simulink model "SURVEY_Simulations"  (R2021b)
settings: Solver=ode4  StartTime=0.0  StopTime=60  FixedStep=1e-3  RelTol=1e-3
(part 1 of 2)
settings Model: Creator=hellb  LastModifiedBy=hellb
settings SolverCC: ZeroCrossAlgorithm=Adaptive
settings DebuggingCC: IgnoredZcDiagnostic=none

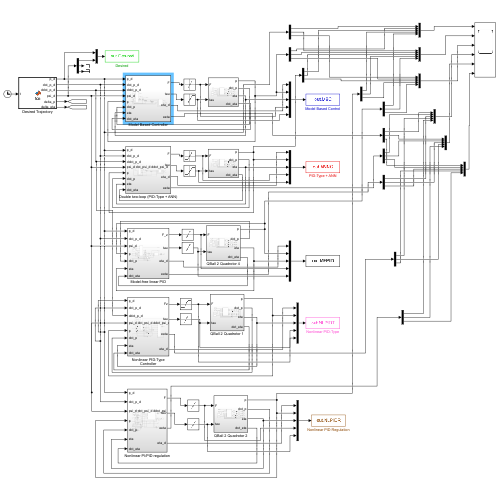
[thumbnail: Simulink's stored preview of the top-level diagram]
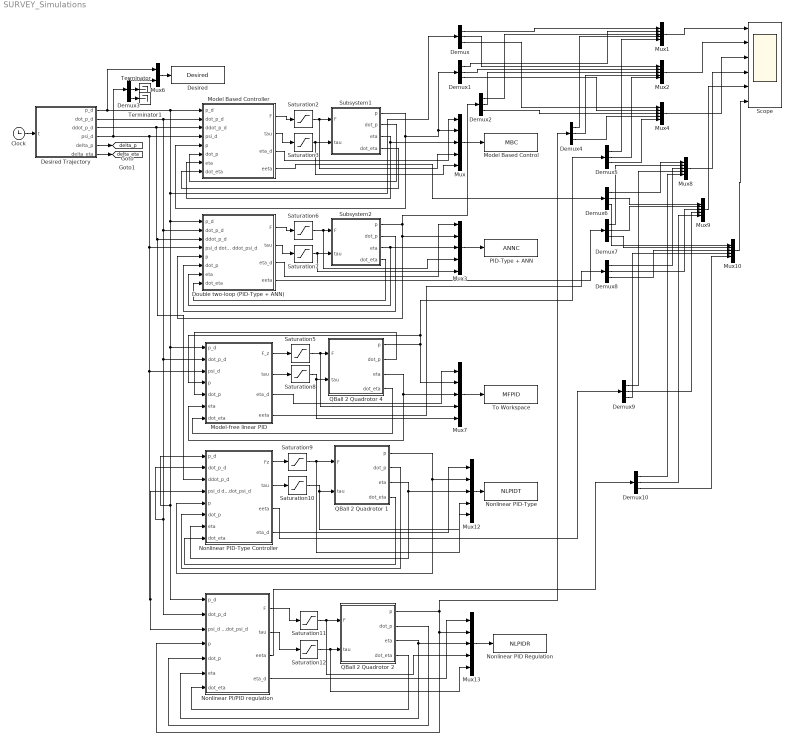
== system SURVEY_Simulations ==
  Clock : Clock
  Demux{,1..10} (11 alike) : Demux  Outputs=3
  Desired : ToWorkspace  VariableName=Desired  SaveFormat=Structure With Time  SampleTime=-1
  Desired Trajectory : MATLAB Function  TreatAsAtomicUnit=on
  Double two-loop (PID-Type + ANN) : Subsystem
  Model Based Control : ToWorkspace  VariableName=MBC  SaveFormat=Structure With Time  SampleTime=-1
  Model Based Controller : Subsystem
  Model-free linear PID : Subsystem
  Mux{,1..4,7..10,12..13} (11 alike) : Mux  Inputs=5
  Mux6 : Mux  Inputs=2
  Nonlinear PI/PID regulation : Subsystem
  Nonlinear PID Regulation : ToWorkspace  VariableName=NLPIDR  SaveFormat=Structure With Time  SampleTime=-1
  Nonlinear PID-Type : ToWorkspace  VariableName=NLPIDT  SaveFormat=Structure With Time  SampleTime=-1
  Nonlinear PID-Type Controller : Subsystem
  PID-Type + ANN : ToWorkspace  VariableName=ANNC  SaveFormat=Structure With Time  SampleTime=-1
  QBall 2 Quadrotor 1 : Subsystem
  QBall 2 Quadrotor 2 : Subsystem
  QBall 2 Quadrotor 4 : Subsystem
  Saturation{3,7..8,10,12} (5 alike) : Saturate  UpperLimit=1.72  LowerLimit=-1.72
  Saturation{2,5..6,9,11} (5 alike) : Saturate  UpperLimit=34.4  LowerLimit=0
  Scope : Scope  NumInputPorts=6
  Subsystem1 : Subsystem
  Subsystem2 : Subsystem
  Terminator : Terminator
  Terminator1 : Terminator
  To Workspace : ToWorkspace  VariableName=MFPID  SaveFormat=Structure With Time  SampleTime=-1
  tag scope: delta_eta=global, delta_p=global
  wires:
  Demux1/3 -> Mux4/2
  Demux3/2 -> Terminator/1
  Subsystem1/2(dot_p) -> Model Based Controller/6(dot_p)
  Demux3/1 -> Mux6/2
  Demux4/3 -> Mux4/4
  Demux4/1 -> Mux1/4
  Demux4/2 -> Mux2/4
  Demux3/3 -> Terminator1/1
  Desired Trajectory/2(dot_p_d) -> Nonlinear PI/PID regulation/2(dot_p_d), Nonlinear PID-Type Controller/2(dot_p_d), Model-free linear PID/2(dot_p_d), Double two-loop (PID-Type + ANN)/2(dot_p_d), Model Based Controller/2(dot_p_d)
  Demux1/2 -> Mux2/2
  Mux6/1 -> Desired/1
  Subsystem2/1(p) -> Demux2/1, Mux3/2, Double two-loop (PID-Type + ANN)/5(p)
  Desired Trajectory/5(delta_p) -> [delta_p]
  Demux/2 -> Mux2/1
  Mux3/1 -> PID-Type + ANN/1
  Mux4/1 -> Scope/3
  Demux2/3 -> Mux4/3
  Desired Trajectory/4(psi_d) -> Nonlinear PI/PID regulation/3(psi_d dot_psi_d ddot_psi_d), Nonlinear PID-Type Controller/4(psi_d dot_psi_d ddot_psi_d), Model-free linear PID/3(psi_d), Double two-loop (PID-Type + ANN)/4(psi_d dot_psi_d ddot_psi_d), Model Based Controller/4(psi_d), Demux3/1
  Double two-loop (PID-Type + ANN)/1(F) -> Saturation6/1
  Model Based Controller/3(eta_d) -> Mux/1
  Mux1/1 -> Scope/1
  Demux/1 -> Mux1/1
  Demux2/2 -> Mux2/3
  Demux2/1 -> Mux1/3
  Model Based Controller/2(tau) -> Saturation3/1
  Desired Trajectory/1(p_d) -> Nonlinear PI/PID regulation/1(p_d), Nonlinear PID-Type Controller/1(p_d), Model-free linear PID/1(p_d), Double two-loop (PID-Type + ANN)/1(p_d), Demux/1, Model Based Controller/1(p_d), Mux6/1
  Subsystem1/1(p) -> Model Based Controller/5(p), Demux1/1, Mux/2
  Subsystem1/4(dot_eta) -> Model Based Controller/8(dot_eta)
  Saturation7/1 -> Subsystem2/2(tau), Mux3/5
  Demux1/1 -> Mux1/2
  Saturation6/1 -> Subsystem2/1(F), Mux3/4
  Subsystem2/2(dot_p) -> Double two-loop (PID-Type + ANN)/6(dot_p)
  Mux/1 -> Model Based Control/1
  Desired Trajectory/3(ddot_p_d) -> Nonlinear PID-Type Controller/3(ddot_p_d), Double two-loop (PID-Type + ANN)/3(ddot_p_d), Model Based Controller/3(ddot_p_d)
  Subsystem1/3(eta) -> Mux/3, Model Based Controller/7(eta)
  Demux/3 -> Mux4/1
  Model Based Controller/1(F) -> Saturation2/1
  Double two-loop (PID-Type + ANN)/3(eta_d) -> Mux3/1
  Double two-loop (PID-Type + ANN)/2(tau) -> Saturation7/1
  Mux2/1 -> Scope/2
  Saturation3/1 -> Mux/5, Subsystem1/2(tau)
  Subsystem2/3(eta) -> Mux3/3, Double two-loop (PID-Type + ANN)/7(eta)
  Desired Trajectory/6(delta_eta) -> [delta_eta]
  Clock/1 -> Desired Trajectory/1(t)
  Subsystem2/4(dot_eta) -> Double two-loop (PID-Type + ANN)/8(dot_eta)
  Model-free linear PID/1(F_z) -> Saturation5/1
  Saturation5/1 -> Mux7/4, QBall 2 Quadrotor 4/1(F)
  QBall 2 Quadrotor 4/4(dot_eta) -> Model-free linear PID/7(dot_eta)
  QBall 2 Quadrotor 4/3(eta) -> Mux7/3, Model-free linear PID/6(eta)
  QBall 2 Quadrotor 4/2(dot_p) -> Model-free linear PID/5(dot_p)
  QBall 2 Quadrotor 4/1(p) -> Mux7/2, Demux5/1, Model-free linear PID/4(p)
  Saturation2/1 -> Mux/4, Subsystem1/1(F)
  Saturation10/1 -> Mux12/5, QBall 2 Quadrotor 1/2(tau)
  Saturation9/1 -> QBall 2 Quadrotor 1/1(F), Mux12/4
  Nonlinear PID-Type Controller/1(Fz) -> Saturation9/1
  Nonlinear PID-Type Controller/2(tau) -> Saturation10/1
  Demux5/1 -> Mux1/5
  Demux5/2 -> Mux2/5
  Demux5/3 -> Mux4/5
  QBall 2 Quadrotor 1/1(p) -> Mux12/2, Nonlinear PID-Type Controller/5(p)
  QBall 2 Quadrotor 1/2(dot_p) -> Nonlinear PID-Type Controller/6(dot_p)
  QBall 2 Quadrotor 1/3(eta) -> Nonlinear PID-Type Controller/7(eta), Mux12/3
  QBall 2 Quadrotor 1/4(dot_eta) -> Nonlinear PID-Type Controller/8(dot_eta)
  Saturation11/1 -> Mux13/4, QBall 2 Quadrotor 2/1(F)
  Saturation12/1 -> Mux13/5, QBall 2 Quadrotor 2/2(tau)
  Nonlinear PI/PID regulation/1(F) -> Saturation11/1
  Nonlinear PI/PID regulation/2(tau) -> Saturation12/1
  QBall 2 Quadrotor 2/1(p) -> Mux13/2, Nonlinear PI/PID regulation/4(p), Demux4/1
  QBall 2 Quadrotor 2/4(dot_eta) -> Nonlinear PI/PID regulation/7(dot_eta)
  QBall 2 Quadrotor 2/3(eta) -> Mux13/3, Nonlinear PI/PID regulation/6(eta)
  QBall 2 Quadrotor 2/2(dot_p) -> Nonlinear PI/PID regulation/5(dot_p)
  Mux9/1 -> Scope/5
  Mux8/1 -> Scope/4
  Mux10/1 -> Scope/6
  Demux6/1 -> Mux8/1
  Demux6/2 -> Mux9/1
  Demux6/3 -> Mux10/1
  Model Based Controller/4(eeta) -> Demux6/1
  Demux7/1 -> Mux8/2
  Demux7/2 -> Mux9/2
  Demux7/3 -> Mux10/2
  Double two-loop (PID-Type + ANN)/4(eeta) -> Demux7/1
  Demux8/1 -> Mux8/3
  Demux8/2 -> Mux9/3
  Demux8/3 -> Mux10/3
  Nonlinear PID-Type Controller/3(eeta) -> Demux9/1
  Demux9/1 -> Mux8/4
  Demux9/2 -> Mux9/4
  Demux9/3 -> Mux10/4
  Nonlinear PI/PID regulation/3(eeta) -> Demux10/1
  Demux10/1 -> Mux8/5
  Demux10/2 -> Mux9/5
  Demux10/3 -> Mux10/5
  Model-free linear PID/3(eta_d) -> Mux7/1
  Nonlinear PID-Type Controller/4(eta_d) -> Mux12/1
  Mux13/1 -> Nonlinear PID Regulation/1
  Nonlinear PI/PID regulation/4(eta_d) -> Mux13/1
  Mux7/1 -> To Workspace/1
  Saturation8/1 -> Mux7/5, QBall 2 Quadrotor 4/2(tau)
  Model-free linear PID/2(tau) -> Saturation8/1
  Mux12/1 -> Nonlinear PID-Type/1
  Model-free linear PID/4(eeta) -> Demux8/1

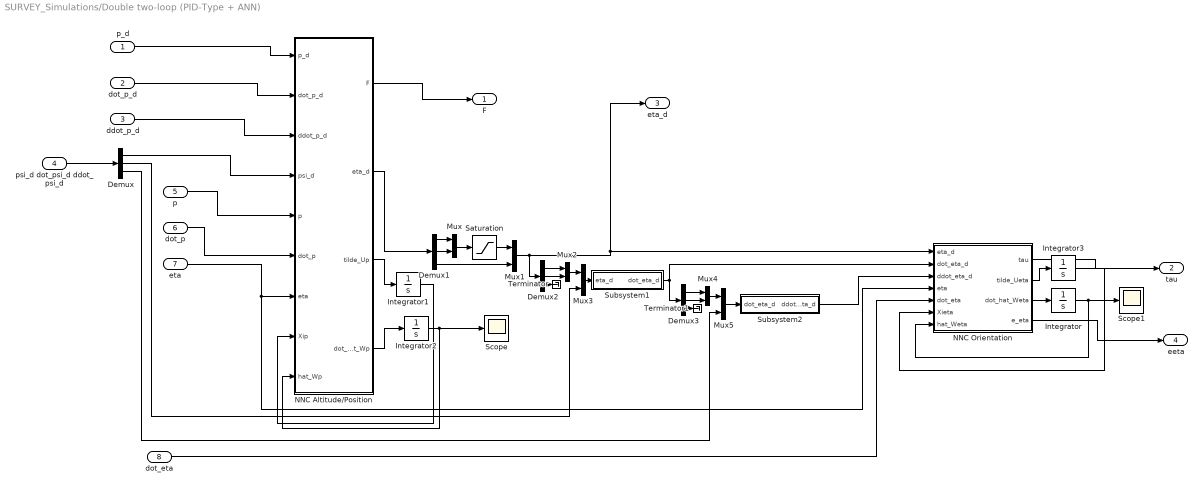
== system SURVEY_Simulations/Double two-loop (PID-Type + ANN) ==
  p_d : Inport
  dot_p_d : Inport  Port=2
  ddot_p_d : Inport  Port=3
  psi_d dot_psi_d ddot_psi_d : Inport  Port=4
  p : Inport  Port=5
  dot_p : Inport  Port=6
  eta : Inport  Port=7
  dot_eta : Inport  Port=8
  Demux{,1..3} (4 alike) : Demux  Outputs=3
  Integrator : Integrator  InitialCondition=zeros(10,3)
  Integrator1 : Integrator  InitialCondition=[0;0;0]
  Integrator2 : Integrator  InitialCondition=zeros(10,3)
  Integrator3 : Integrator  InitialCondition=[0;0;0]
  Mux{,1..5} (6 alike) : Mux  Inputs=2
  NNC Altitude/Position : MATLAB Function  TreatAsAtomicUnit=on
  NNC Orientation : MATLAB Function  TreatAsAtomicUnit=on
  Saturation : Saturate  UpperLimit=20*pi/180  LowerLimit=-20*pi/180
  Scope : Scope
  Scope1 : Scope
  Subsystem1 : Subsystem
  Subsystem2 : Subsystem
  Terminator : Terminator
  Terminator1 : Terminator
  F : Outport
  tau : Outport  Port=2
  eta_d : Outport  Port=3
  eeta : Outport  Port=4
  wires:
  NNC Altitude/Position/4(dot_hat_Wp) -> Integrator2/1
  Integrator/1 -> Scope1/1, NNC Orientation/7(hat_Weta)
  NNC Orientation/3(dot_hat_Weta) -> Integrator/1
  Integrator2/1 -> Scope/1, NNC Altitude/Position/9(hat_Wp)
  psi_d dot_psi_d ddot_psi_d/1 -> Demux/1
  Demux3/3 -> Terminator1/1
  Mux4/1 -> Mux5/1
  Demux3/1 -> Mux4/1
  Demux3/2 -> Mux4/2
  Demux/3 -> Mux5/2
  Demux/2 -> Mux3/2
  NNC Altitude/Position/2(eta_d) -> Demux1/1
  Demux1/1 -> Mux/1
  Demux2/2 -> Mux2/2
  Mux3/1 -> Subsystem1/1(eta_d)
  Demux1/3 -> Mux1/2
  Mux2/1 -> Mux3/1
  Demux2/3 -> Terminator/1
  Saturation/1 -> Mux1/1
  Demux1/2 -> Mux/2
  Mux5/1 -> Subsystem2/1(dot_eta_d)
  Demux2/1 -> Mux2/1
  Subsystem1/1(dot_eta_d) -> NNC Orientation/2(dot_eta_d), Demux3/1
  Mux1/1 -> NNC Orientation/1(eta_d), eta_d/1, Demux2/1
  Mux/1 -> Saturation/1
  Subsystem2/1(ddot_eta_d) -> NNC Orientation/3(ddot_eta_d)
  Demux/1 -> NNC Altitude/Position/4(psi_d)
  NNC Orientation/1(tau) -> tau/1
  NNC Altitude/Position/1(F) -> F/1
  dot_p_d/1 -> NNC Altitude/Position/2(dot_p_d)
  p_d/1 -> NNC Altitude/Position/1(p_d)
  eta/1 -> NNC Orientation/4(eta), NNC Altitude/Position/7(eta)
  p/1 -> NNC Altitude/Position/5(p)
  dot_p/1 -> NNC Altitude/Position/6(dot_p)
  dot_eta/1 -> NNC Orientation/5(dot_eta)
  ddot_p_d/1 -> NNC Altitude/Position/3(ddot_p_d)
  NNC Orientation/4(e_eta) -> eeta/1
  NNC Altitude/Position/3(tilde_Up) -> Integrator1/1
  Integrator1/1 -> NNC Altitude/Position/8(Xip)
  NNC Orientation/2(tilde_Ueta) -> Integrator3/1
  Integrator3/1 -> NNC Orientation/6(Xieta)

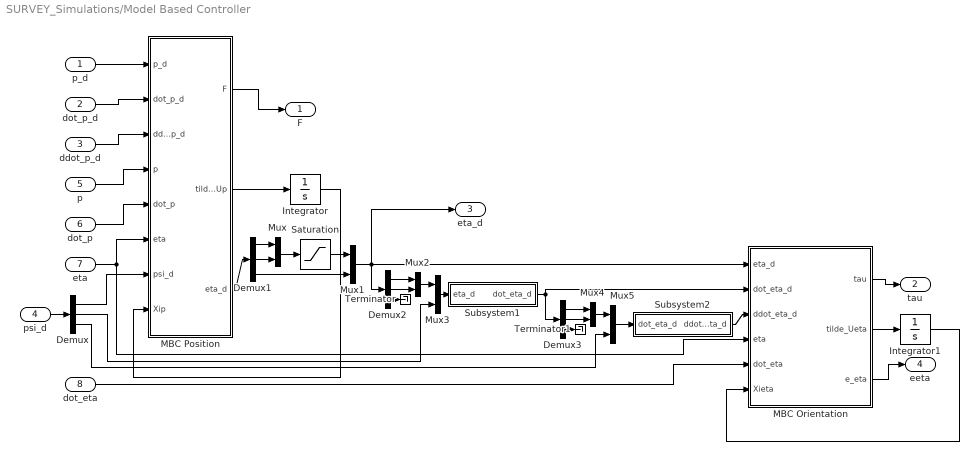
== system SURVEY_Simulations/Model Based Controller ==
  p_d : Inport
  dot_p_d : Inport  Port=2
  ddot_p_d : Inport  Port=3
  psi_d : Inport  Port=4
  p : Inport  Port=5
  dot_p : Inport  Port=6
  eta : Inport  Port=7
  dot_eta : Inport  Port=8
  Demux{,1..3} (4 alike) : Demux  Outputs=3
  Integrator : Integrator  InitialCondition=[0;0;0]
  Integrator1 : Integrator  InitialCondition=[0;0;0]
  MBC Orientation : MATLAB Function  TreatAsAtomicUnit=on
  MBC Position : MATLAB Function  TreatAsAtomicUnit=on
  Mux{,1..5} (6 alike) : Mux  Inputs=2
  Saturation : Saturate  UpperLimit=20*pi/180  LowerLimit=-20*pi/180
  Subsystem1 : Subsystem
  Subsystem2 : Subsystem
  Terminator : Terminator
  Terminator1 : Terminator
  F : Outport
  tau : Outport  Port=2
  eta_d : Outport  Port=3
  eeta : Outport  Port=4
  wires:
  psi_d/1 -> Demux/1
  Subsystem1/1(dot_eta_d) -> Demux3/1, MBC Orientation/2(dot_eta_d)
  Subsystem2/1(ddot_eta_d) -> MBC Orientation/3(ddot_eta_d)
  MBC Position/1(F) -> F/1
  eta/1 -> MBC Orientation/4(eta), MBC Position/6(eta)
  ddot_p_d/1 -> MBC Position/3(ddot_p_d)
  MBC Orientation/1(tau) -> tau/1
  p/1 -> MBC Position/4(p)
  dot_p/1 -> MBC Position/5(dot_p)
  p_d/1 -> MBC Position/1(p_d)
  dot_eta/1 -> MBC Orientation/5(dot_eta)
  dot_p_d/1 -> MBC Position/2(dot_p_d)
  Mux1/1 -> Demux2/1, eta_d/1, MBC Orientation/1(eta_d)
  Demux/1 -> MBC Position/7(psi_d)
  MBC Position/3(eta_d) -> Demux1/1
  Demux1/2 -> Mux/2
  Demux1/1 -> Mux/1
  Mux/1 -> Saturation/1
  Saturation/1 -> Mux1/1
  Demux1/3 -> Mux1/2
  Demux2/2 -> Mux2/2
  Demux2/1 -> Mux2/1
  Mux2/1 -> Mux3/1
  Mux3/1 -> Subsystem1/1(eta_d)
  Demux/2 -> Mux3/2
  Demux2/3 -> Terminator/1
  Demux3/2 -> Mux4/2
  Mux5/1 -> Subsystem2/1(dot_eta_d)
  Mux4/1 -> Mux5/1
  Demux3/1 -> Mux4/1
  Demux3/3 -> Terminator1/1
  Demux/3 -> Mux5/2
  MBC Orientation/3(e_eta) -> eeta/1
  MBC Position/2(tilde_Up) -> Integrator/1
  Integrator/1 -> MBC Position/8(Xip)
  MBC Orientation/2(tilde_Ueta) -> Integrator1/1
  Integrator1/1 -> MBC Orientation/6(Xieta)

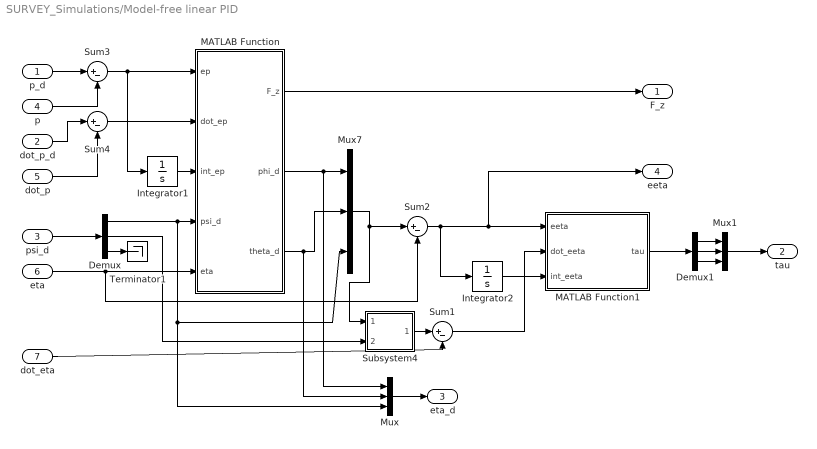
== system SURVEY_Simulations/Model-free linear PID ==
  p_d : Inport
  dot_p_d : Inport  Port=2
  psi_d : Inport  Port=3
  p : Inport  Port=4
  dot_p : Inport  Port=5
  eta : Inport  Port=6
  dot_eta : Inport  Port=7
  Demux : Demux  Outputs=3
  Demux1 : Demux  Outputs=3
  Integrator1 : Integrator  InitialCondition=[0;0;0]
  Integrator2 : Integrator  InitialCondition=[0;0;0]
  MATLAB Function : MATLAB Function  TreatAsAtomicUnit=on
  MATLAB Function1 : MATLAB Function  TreatAsAtomicUnit=on
  Mux : Mux  Inputs=3
  Mux1 : Mux  Inputs=3
  Mux7 : Mux  Inputs=3
  Subsystem4 : Subsystem
  Sum{1..4} (4 alike) : Sum  Inputs=|+-
  Terminator1 : Terminator
  F_z : Outport
  tau : Outport  Port=2
  eta_d : Outport  Port=3
  eeta : Outport  Port=4
  wires:
  dot_eta/1 -> Sum1/2
  MATLAB Function/3(theta_d) -> Mux/2, Mux7/2
  Sum1/1 -> MATLAB Function1/2(dot_eeta)
  Mux7/1 -> Subsystem4/1(eta_d(1,2)), Sum2/1
  MATLAB Function/2(phi_d) -> Mux/1, Mux7/1
  Integrator2/1 -> MATLAB Function1/3(int_eeta)
  eta/1 -> MATLAB Function/5(eta), Sum2/2
  MATLAB Function/1(F_z) -> F_z/1
  Subsystem4/1(dot_eta_d) -> Sum1/1
  Sum2/1 -> Integrator2/1, eeta/1, MATLAB Function1/1(eeta)
  p_d/1 -> Sum3/1
  Sum3/1 -> Integrator1/1, MATLAB Function/1(ep)
  p/1 -> Sum3/2
  dot_p/1 -> Sum4/2
  dot_p_d/1 -> Sum4/1
  Sum4/1 -> MATLAB Function/2(dot_ep)
  Integrator1/1 -> MATLAB Function/3(int_ep)
  psi_d/1 -> Demux/1
  Demux/1 -> Mux/3, Mux7/3, MATLAB Function/4(psi_d)
  Demux/2 -> Subsystem4/2(dot_psi_d)
  Demux/3 -> Terminator1/1
  Mux/1 -> eta_d/1
  MATLAB Function1/1(tau) -> Demux1/1
  Demux1/1 -> Mux1/1
  Demux1/2 -> Mux1/2
  Demux1/3 -> Mux1/3
  Mux1/1 -> tau/1

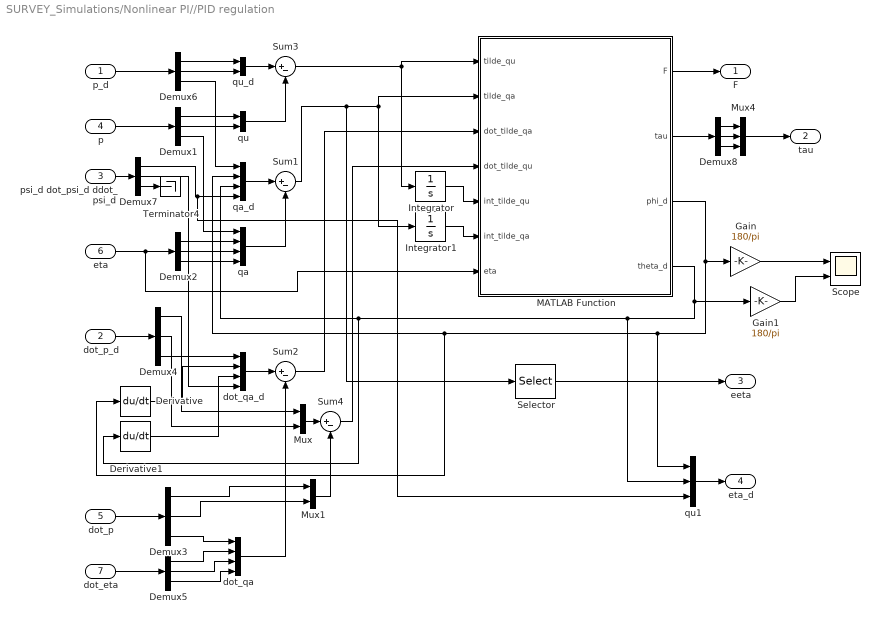
== system SURVEY_Simulations/Nonlinear PI//PID regulation ==
  p_d : Inport
  dot_p_d : Inport  Port=2
  psi_d dot_psi_d ddot_psi_d : Inport  Port=3
  p : Inport  Port=4
  dot_p : Inport  Port=5
  eta : Inport  Port=6
  dot_eta : Inport  Port=7
  Demux{1..8} (8 alike) : Demux  Outputs=3
  Derivative : Derivative
  Derivative1 : Derivative
  Gain : Gain  Gain=180/pi
  Gain1 : Gain  Gain=180/pi
  Integrator : Integrator  InitialCondition=[0; 0]
  Integrator1 : Integrator  InitialCondition=[0; 0; 0; 0]
  MATLAB Function : MATLAB Function  TreatAsAtomicUnit=on
  Mux : Mux  Inputs=2
  Mux1 : Mux  Inputs=2
  Mux4 : Mux  Inputs=3
  Scope : Scope  NumInputPorts=2
  Selector : Selector  InputPortWidth=4  IndexOptions=Starting index (dialog)  Indices=[2]  OutputSizes=3
  Sum{1..4} (4 alike) : Sum  Inputs=|+-
  Terminator4 : Terminator
  dot_qa : Mux
  dot_qa_d : Mux
  qa : Mux
  qa_d : Mux
  qu : Mux  Inputs=2
  qu1 : Mux  Inputs=3
  qu_d : Mux  Inputs=2
  F : Outport
  tau : Outport  Port=2
  eeta : Outport  Port=3
  eta_d : Outport  Port=4
  wires:
  Demux6/1 -> qu_d/1
  Demux6/3 -> qa_d/1
  MATLAB Function/4(theta_d) -> qu1/2, Derivative1/1, qa_d/3, Gain1/1
  qu_d/1 -> Sum3/1
  Demux7/1 -> qu1/3, qa_d/4
  MATLAB Function/3(phi_d) -> Gain/1, qu1/1, Derivative/1, qa_d/2
  Demux6/2 -> qu_d/2
  qa_d/1 -> Sum1/1
  p_d/1 -> Demux6/1
  MATLAB Function/1(F) -> F/1
  psi_d dot_psi_d ddot_psi_d/1 -> Demux7/1
  p/1 -> Demux1/1
  Demux1/1 -> qu/1
  Demux1/2 -> qu/2
  qu/1 -> Sum3/2
  Sum3/1 -> Integrator/1, MATLAB Function/1(tilde_qu)
  Demux1/3 -> qa/1
  eta/1 -> MATLAB Function/7(eta), Demux2/1
  Demux2/1 -> qa/2
  Demux2/2 -> qa/3
  Demux2/3 -> qa/4
  qa/1 -> Sum1/2
  Sum1/1 -> Selector/1, Integrator1/1, MATLAB Function/2(tilde_qa)
  dot_p_d/1 -> Demux4/1
  Demux4/3 -> dot_qa_d/1
  Demux4/1 -> Mux/1
  Demux4/2 -> Mux/2
  Demux7/2 -> dot_qa_d/4
  Derivative/1 -> dot_qa_d/2
  Derivative1/1 -> dot_qa_d/3
  Demux3/2 -> Mux1/2
  Demux3/1 -> Mux1/1
  dot_p/1 -> Demux3/1
  dot_eta/1 -> Demux5/1
  Demux3/3 -> dot_qa/1
  Demux5/1 -> dot_qa/2
  Demux5/2 -> dot_qa/3
  Demux5/3 -> dot_qa/4
  dot_qa/1 -> Sum2/2
  dot_qa_d/1 -> Sum2/1
  Sum2/1 -> MATLAB Function/3(dot_tilde_qa)
  Integrator/1 -> MATLAB Function/5(int_tilde_qu)
  Integrator1/1 -> MATLAB Function/6(int_tilde_qa)
  Demux7/3 -> Terminator4/1
  Selector/1 -> eeta/1
  qu1/1 -> eta_d/1
  Demux8/3 -> Mux4/3
  Demux8/2 -> Mux4/2
  Demux8/1 -> Mux4/1
  MATLAB Function/2(tau) -> Demux8/1
  Mux4/1 -> tau/1
  Gain/1 -> Scope/1
  Gain1/1 -> Scope/2
  Mux/1 -> Sum4/1
  Mux1/1 -> Sum4/2
  Sum4/1 -> MATLAB Function/4(dot_tilde_qu)

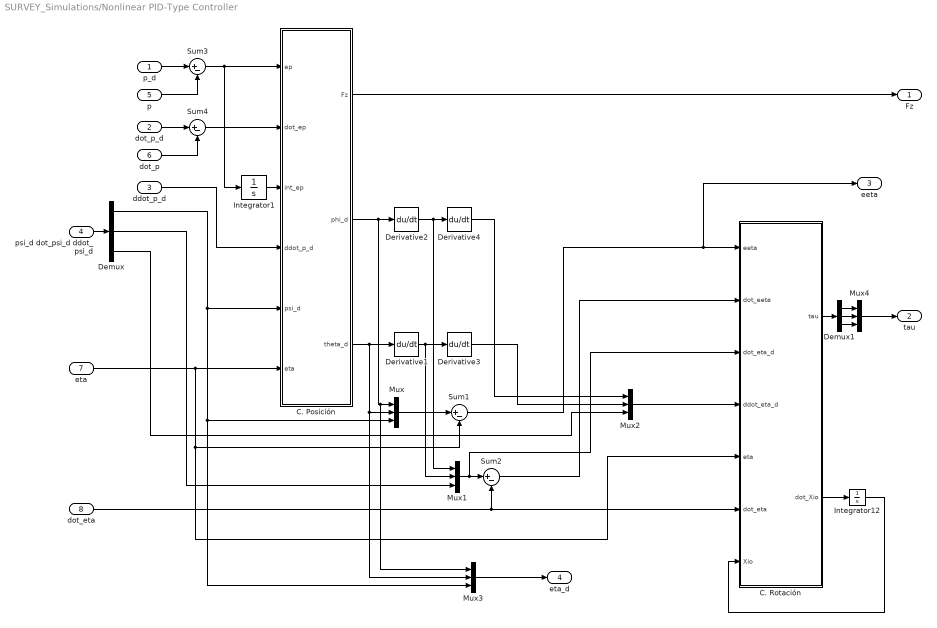
== system SURVEY_Simulations/Nonlinear PID-Type Controller ==
  p_d : Inport
  dot_p_d : Inport  Port=2
  ddot_p_d : Inport  Port=3
  psi_d dot_psi_d ddot_psi_d : Inport  Port=4
  p : Inport  Port=5
  dot_p : Inport  Port=6
  eta : Inport  Port=7
  dot_eta : Inport  Port=8
  C. Posición : MATLAB Function  TreatAsAtomicUnit=on
  C. Rotación : MATLAB Function  TreatAsAtomicUnit=on
  Demux : Demux  Outputs=3
  Demux1 : Demux  Outputs=3
  Derivative{1..4} (4 alike) : Derivative
  Integrator1 : Integrator  InitialCondition=[0;0;0]
  Integrator12 : Integrator  InitialCondition=[0;0;0]
  Mux{,1..4} (5 alike) : Mux  Inputs=3
  Sum{1..4} (4 alike) : Sum  Inputs=|+-
  Fz : Outport
  tau : Outport  Port=2
  eeta : Outport  Port=3
  eta_d : Outport  Port=4
  wires:
  C. Posición/1(Fz) -> Fz/1
  C. Rotación/2(dot_Xio) -> Integrator12/1
  dot_p/1 -> Sum4/2
  Integrator1/1 -> C. Posición/3(int_ep)
  dot_p_d/1 -> Sum4/1
  Demux/3 -> Mux2/3
  p_d/1 -> Sum3/1
  psi_d dot_psi_d ddot_psi_d/1 -> Demux/1
  p/1 -> Sum3/2
  Sum3/1 -> C. Posición/1(ep), Integrator1/1
  Sum4/1 -> C. Posición/2(dot_ep)
  ddot_p_d/1 -> C. Posición/4(ddot_p_d)
  Demux/1 -> Mux/3, Mux3/3, C. Posición/5(psi_d)
  eta/1 -> C. Posición/6(eta), Sum1/2, C. Rotación/5(eta)
  Derivative1/1 -> Derivative3/1, Mux1/2
  Derivative2/1 -> Derivative4/1, Mux1/1
  Mux/1 -> Sum1/1
  Integrator12/1 -> C. Rotación/7(Xio)
  C. Posición/2(phi_d) -> Derivative2/1, Mux3/1, Mux/1
  C. Posición/3(theta_d) -> Derivative1/1, Mux3/2, Mux/2
  Demux/2 -> Mux1/3
  Mux1/1 -> C. Rotación/3(dot_eta_d), Sum2/1
  dot_eta/1 -> Sum2/2, C. Rotación/6(dot_eta)
  Derivative4/1 -> Mux2/1
  Derivative3/1 -> Mux2/2
  Sum1/1 -> eeta/1, C. Rotación/1(eeta)
  Sum2/1 -> C. Rotación/2(dot_eeta)
  Mux2/1 -> C. Rotación/4(ddot_eta_d)
  Mux3/1 -> eta_d/1
  Demux1/1 -> Mux4/1
  Demux1/2 -> Mux4/2
  Demux1/3 -> Mux4/3
  Mux4/1 -> tau/1
  C. Rotación/1(tau) -> Demux1/1

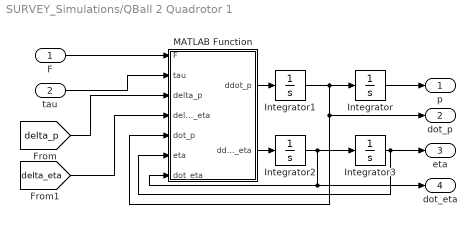
== system SURVEY_Simulations/QBall 2 Quadrotor 1 ==
  F : Inport
  tau : Inport  Port=2
  Integrator : Integrator  InitialCondition=[0;0;0.3]  LimitOutput=on  UpperSaturationLimit=[inf;inf;inf]  LowerSaturationLimit=[-inf;-inf;0.3]
  Integrator1 : Integrator  InitialCondition=[0;0;0]
  Integrator2 : Integrator  InitialCondition=[0;0;0]
  Integrator3 : Integrator  InitialCondition=[0;0;0]  LimitOutput=on  UpperSaturationLimit=[pi/2; pi/2; inf]  LowerSaturationLimit=[-pi/2; -pi/2; -inf]
  MATLAB Function : MATLAB Function  TreatAsAtomicUnit=on
  p : Outport
  dot_p : Outport  Port=2
  eta : Outport  Port=3
  dot_eta : Outport  Port=4
  wires:
  [delta_p] -> MATLAB Function/3(delta_p)
  [delta_eta] -> MATLAB Function/4(delta_eta)
  F/1 -> MATLAB Function/1(F)
  Integrator3/1 -> MATLAB Function/6(eta), eta/1
  Integrator1/1 -> dot_p/1, MATLAB Function/5(dot_p), Integrator/1
  MATLAB Function/2(ddot_eta) -> Integrator2/1
  MATLAB Function/1(ddot_p) -> Integrator1/1
  tau/1 -> MATLAB Function/2(tau)
  Integrator2/1 -> Integrator3/1, dot_eta/1, MATLAB Function/7(dot_eta)
  Integrator/1 -> p/1

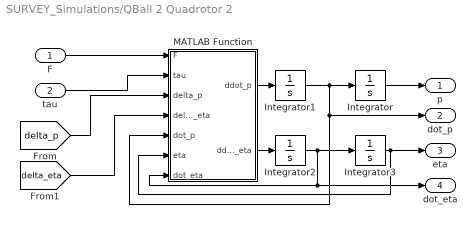
== system SURVEY_Simulations/QBall 2 Quadrotor 2 ==
  F : Inport
  tau : Inport  Port=2
  Integrator : Integrator  InitialCondition=[0;0;0.3]  LimitOutput=on  UpperSaturationLimit=[inf;inf;inf]  LowerSaturationLimit=[-inf;-inf;0.3]
  Integrator1 : Integrator  InitialCondition=[0;0;0]
  Integrator2 : Integrator  InitialCondition=[0;0;0]
  Integrator3 : Integrator  InitialCondition=[0;0;0]  LimitOutput=on  UpperSaturationLimit=[pi/2; pi/2; inf]  LowerSaturationLimit=[-pi/2; -pi/2; -inf]
  MATLAB Function : MATLAB Function  TreatAsAtomicUnit=on
  p : Outport
  dot_p : Outport  Port=2
  eta : Outport  Port=3
  dot_eta : Outport  Port=4
  wires:
  Integrator/1 -> p/1
  Integrator2/1 -> MATLAB Function/7(dot_eta), dot_eta/1, Integrator3/1
  tau/1 -> MATLAB Function/2(tau)
  MATLAB Function/1(ddot_p) -> Integrator1/1
  MATLAB Function/2(ddot_eta) -> Integrator2/1
  Integrator1/1 -> Integrator/1, MATLAB Function/5(dot_p), dot_p/1
  Integrator3/1 -> eta/1, MATLAB Function/6(eta)
  F/1 -> MATLAB Function/1(F)
  [delta_eta] -> MATLAB Function/4(delta_eta)
  [delta_p] -> MATLAB Function/3(delta_p)

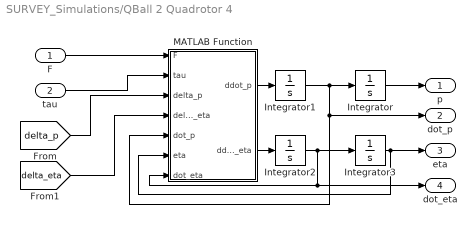
== system SURVEY_Simulations/QBall 2 Quadrotor 4 ==
  F : Inport
  tau : Inport  Port=2
  Integrator : Integrator  InitialCondition=[0;0;0.3]  LimitOutput=on  UpperSaturationLimit=[inf;inf;inf]  LowerSaturationLimit=[-inf;-inf;0.3]
  Integrator1 : Integrator  InitialCondition=[0;0;0]
  Integrator2 : Integrator  InitialCondition=[0;0;0]
  Integrator3 : Integrator  InitialCondition=[0;0;0]  LimitOutput=on  UpperSaturationLimit=[pi/2; pi/2; inf]  LowerSaturationLimit=[-pi/2; -pi/2; -inf]
  MATLAB Function : MATLAB Function  TreatAsAtomicUnit=on
  p : Outport
  dot_p : Outport  Port=2
  eta : Outport  Port=3
  dot_eta : Outport  Port=4
  wires:
  Integrator/1 -> p/1
  Integrator2/1 -> MATLAB Function/7(dot_eta), dot_eta/1, Integrator3/1
  tau/1 -> MATLAB Function/2(tau)
  MATLAB Function/1(ddot_p) -> Integrator1/1
  MATLAB Function/2(ddot_eta) -> Integrator2/1
  Integrator1/1 -> Integrator/1, MATLAB Function/5(dot_p), dot_p/1
  Integrator3/1 -> eta/1, MATLAB Function/6(eta)
  F/1 -> MATLAB Function/1(F)
  [delta_eta] -> MATLAB Function/4(delta_eta)
  [delta_p] -> MATLAB Function/3(delta_p)

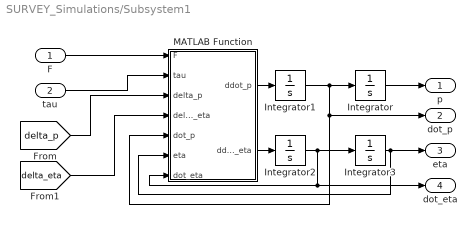
== system SURVEY_Simulations/Subsystem1 ==
  F : Inport
  tau : Inport  Port=2
  Integrator : Integrator  InitialCondition=[0;0;0.3]  LimitOutput=on  UpperSaturationLimit=[inf;inf;inf]  LowerSaturationLimit=[-inf;-inf;0.3]
  Integrator1 : Integrator  InitialCondition=[0;0;0]
  Integrator2 : Integrator  InitialCondition=[0;0;0]
  Integrator3 : Integrator  InitialCondition=[0;0;0]  LimitOutput=on  UpperSaturationLimit=[pi/2; pi/2; inf]  LowerSaturationLimit=[-pi/2; -pi/2; -inf]
  MATLAB Function : MATLAB Function  TreatAsAtomicUnit=on
  p : Outport
  dot_p : Outport  Port=2
  eta : Outport  Port=3
  dot_eta : Outport  Port=4
  wires:
  [delta_p] -> MATLAB Function/3(delta_p)
  [delta_eta] -> MATLAB Function/4(delta_eta)
  F/1 -> MATLAB Function/1(F)
  Integrator3/1 -> MATLAB Function/6(eta), eta/1
  Integrator1/1 -> dot_p/1, MATLAB Function/5(dot_p), Integrator/1
  MATLAB Function/2(ddot_eta) -> Integrator2/1
  MATLAB Function/1(ddot_p) -> Integrator1/1
  tau/1 -> MATLAB Function/2(tau)
  Integrator2/1 -> Integrator3/1, dot_eta/1, MATLAB Function/7(dot_eta)
  Integrator/1 -> p/1

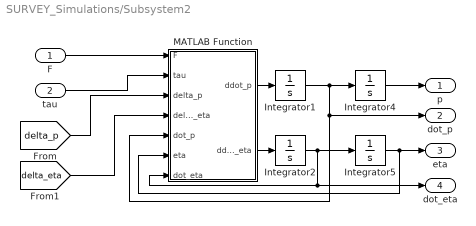
== system SURVEY_Simulations/Subsystem2 ==
  F : Inport
  tau : Inport  Port=2
  Integrator1 : Integrator  InitialCondition=[0;0;0]
  Integrator2 : Integrator  InitialCondition=[0;0;0]
  Integrator4 : Integrator  InitialCondition=[0;0;0.3]  LimitOutput=on  UpperSaturationLimit=[inf;inf;inf]  LowerSaturationLimit=[-inf;-inf;0.3]
  Integrator5 : Integrator  InitialCondition=[0;0;0]  LimitOutput=on  UpperSaturationLimit=[pi/2; pi/2; inf]  LowerSaturationLimit=[-pi/2; -pi/2; -inf]
  MATLAB Function : MATLAB Function  TreatAsAtomicUnit=on
  p : Outport
  dot_p : Outport  Port=2
  eta : Outport  Port=3
  dot_eta : Outport  Port=4
  wires:
  [delta_p] -> MATLAB Function/3(delta_p)
  [delta_eta] -> MATLAB Function/4(delta_eta)
  F/1 -> MATLAB Function/1(F)
  MATLAB Function/2(ddot_eta) -> Integrator2/1
  MATLAB Function/1(ddot_p) -> Integrator1/1
  tau/1 -> MATLAB Function/2(tau)
  Integrator4/1 -> p/1
  Integrator5/1 -> eta/1, MATLAB Function/6(eta)
  Integrator1/1 -> Integrator4/1, dot_p/1, MATLAB Function/5(dot_p)
  Integrator2/1 -> Integrator5/1, dot_eta/1, MATLAB Function/7(dot_eta)

== system SURVEY_Simulations/Double two-loop (PID-Type + ANN)/Subsystem1 ==
  eta_d : Inport
  Demux : Demux  Outputs=3
  Mux : Mux  Inputs=3
  Transfer Fcn : TransferFcn  Numerator=[20 0]  Denominator=[1 20]
  Transfer Fcn1 : TransferFcn  Numerator=[20 0]  Denominator=[1 20]
  dot_eta_d : Outport
  wires:
  Demux/2 -> Transfer Fcn1/1
  Demux/3 -> Mux/3
  Demux/1 -> Transfer Fcn/1
  Transfer Fcn/1 -> Mux/1
  Transfer Fcn1/1 -> Mux/2
  Mux/1 -> dot_eta_d/1
  eta_d/1 -> Demux/1

== system SURVEY_Simulations/Double two-loop (PID-Type + ANN)/Subsystem2 ==
  dot_eta_d : Inport
  Demux : Demux  Outputs=3
  Mux : Mux  Inputs=3
  Transfer Fcn : TransferFcn  Numerator=[20 0]  Denominator=[1 20]
  Transfer Fcn1 : TransferFcn  Numerator=[20 0]  Denominator=[1 20]
  ddot_eta_d : Outport
  wires:
  Demux/3 -> Mux/3
  Transfer Fcn1/1 -> Mux/2
  Demux/2 -> Transfer Fcn1/1
  Demux/1 -> Transfer Fcn/1
  Transfer Fcn/1 -> Mux/1
  dot_eta_d/1 -> Demux/1
  Mux/1 -> ddot_eta_d/1

== system SURVEY_Simulations/Model Based Controller/Subsystem1 ==
  eta_d : Inport
  Demux : Demux  Outputs=3
  Mux : Mux  Inputs=3
  Transfer Fcn : TransferFcn  Numerator=[20 0]  Denominator=[1 20]
  Transfer Fcn1 : TransferFcn  Numerator=[20 0]  Denominator=[1 20]
  dot_eta_d : Outport
  wires:
  Demux/2 -> Transfer Fcn1/1
  Demux/3 -> Mux/3
  Demux/1 -> Transfer Fcn/1
  Transfer Fcn/1 -> Mux/1
  Transfer Fcn1/1 -> Mux/2
  Mux/1 -> dot_eta_d/1
  eta_d/1 -> Demux/1

== system SURVEY_Simulations/Model Based Controller/Subsystem2 ==
  dot_eta_d : Inport
  Demux : Demux  Outputs=3
  Mux : Mux  Inputs=3
  Transfer Fcn : TransferFcn  Numerator=[20 0]  Denominator=[1 20]
  Transfer Fcn1 : TransferFcn  Numerator=[20 0]  Denominator=[1 20]
  ddot_eta_d : Outport
  wires:
  Demux/3 -> Mux/3
  Transfer Fcn1/1 -> Mux/2
  Demux/2 -> Transfer Fcn1/1
  Demux/1 -> Transfer Fcn/1
  Transfer Fcn/1 -> Mux/1
  dot_eta_d/1 -> Demux/1
  Mux/1 -> ddot_eta_d/1

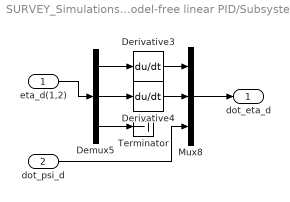
== system SURVEY_Simulations/Model-free linear PID/Subsystem4 ==
  eta_d(1,2) : Inport
  dot_psi_d : Inport  Port=2
  Demux5 : Demux  Outputs=3
  Derivative3 : Derivative
  Derivative4 : Derivative
  Mux8 : Mux  Inputs=3
  Terminator : Terminator
  dot_eta_d : Outport
  wires:
  Demux5/1 -> Derivative3/1
  Derivative3/1 -> Mux8/1
  Mux8/1 -> dot_eta_d/1
  eta_d(1,2)/1 -> Demux5/1
  Derivative4/1 -> Mux8/2
  Demux5/2 -> Derivative4/1
  dot_psi_d/1 -> Mux8/3
  Demux5/3 -> Terminator/1

== matlab function SURVEY_Simulations/Nonlinear PID-Type Controller/C. Rotación ==
  data: eeta input; dot_eeta input; dot_eta_d input; tau output; ddot_eta_d input; eta input; dot_eta input; dot_Xio output; Xio input
function [tau,dot_Xio] = fcn(eeta,dot_eeta,dot_eta_d,ddot_eta_d,eta,dot_eta,Xio)
%-------------
phi   = eta(1);
theta = eta(2);
dot_phi   = dot_eta(1);
dot_theta = dot_eta(2);
dot_psi   = dot_eta(3);
%--------Gains
Kpo = 3*diag([0.125, 0.125, 0.217]);
Kdo = 1.5*diag([0.6, 0.6, 1.0]);
Kio = 2*diag([0.01, 0.01, 0.01]);
Ko  = 5*diag([0.09 0.09 0.09]);
alpha = 0.05;
beta  = 1;
sigma = 20;
%------------------------------------------------
Ixx = 0.00749;
Iyy = 0.00978;
Izz = 0.05130;
I   = diag([Ixx Iyy Izz]);
%-----------------------------------------------------
W = [1 sin(phi)*tan(theta) cos(phi)*tan(theta);
      0     cos(phi)            -sin(phi);
      0 sin(phi)/cos(theta) cos(phi)/cos(theta)];
%--------Transpuesta Inversa de W(n)
InvWnt = [     1              0                 0;
               0           cos(phi)         -sin(phi);
          -sin(theta) cos(theta)*sin(phi) cos(theta)*cos(phi)];
%--------Inversa de W(n)
InvWn = [1     0        -sin(theta);
         0  cos(phi) cos(theta)*sin(phi);
         0 -sin(phi) cos(theta)*cos(phi)];
%-----------Wp(n)
Wnp = [0 cos(phi)*sin(theta)*dot_phi/cos(theta) + sin(phi)*dot_theta/(cos(theta)^2) -sin(phi)*sin(theta)*dot_phi/cos(theta) + cos(phi)*dot_theta/(cos(theta)^2);
         0 -sin(phi)*dot_phi                                        -cos(phi)*dot_phi;
         0 (cos(phi)*cos(theta)*dot_phi+sin(phi)*sin(theta)*dot_theta)/(cos(theta)^2) (-sin(phi)*cos(theta)*dot_phi+cos(phi)*sin(theta)*dot_theta)/(cos(theta)^2) ];
%------producto de W(n)*np y seleccionado para skew symmetric matrix      
SWnnp = [                  0                       -(dot_psi*cos(theta)*cos(phi)-dot_phi*sin(phi)) dot_theta*cos(phi)+dot_psi*cos(theta)*sin(phi);
           dot_psi*cos(theta)*cos(phi)-dot_phi*sin(phi)                        0                            -(dot_phi-dot_psi*sin(theta));
         -(dot_theta*cos(phi)+dot_psi*cos(theta)*sin(phi))              dot_phi-dot_psi*sin(theta)                             0];
%----------------------------------------------
Ho = InvWnt*I*InvWn;
Co = InvWnt*(SWnnp*I-I*InvWn*Wnp)*InvWn;
%------------------------------------------------
dot_Xio = -Ko*Xio + alpha*tanh(sigma*eeta) + beta*dot_eeta;
%------------------------------------------------
tau = W'*(Ho*ddot_eta_d + Co*dot_eta_d + Kpo*tanh(sigma*eeta) + Kio*Xio + Kdo*dot_eeta);

== matlab function SURVEY_Simulations/Model-free linear PID/MATLAB Function ==
  data: ep input; F_z output; dot_ep input; int_ep input; psi_d input; eta input; phi_d output; theta_d output
function [F_z, phi_d, theta_d]  = fcn(ep, dot_ep, int_ep, psi_d, eta)

Kpp = diag([12 12 95]);
Kdp = diag([5 5 35]);
Kip = diag([5 5 25]);

phi   = eta(1);
theta = eta(2);

f_p     = Kpp*ep + Kdp*dot_ep + Kip*int_ep;
theta_d = atan((f_p(2)*sin(psi_d) + f_p(1)*cos(psi_d))/f_p(3));
phi_d   = atan(cos(theta_d)*(f_p(1)*sin(psi_d) - f_p(2)*cos(psi_d))/f_p(3));
F_z     = f_p(3)/(cos(theta)*cos(phi));

== matlab function SURVEY_Simulations/Double two-loop (PID-Type + ANN)/NNC Altitude//Position ==
  data: p_d input; F output; dot_p_d input; ddot_p_d input; psi_d input; p input; dot_p input; eta input; Xip input; eta_d output; tilde_Up output; dot_hat_Wp output; hat_Wp input
function [F, eta_d, tilde_Up, dot_hat_Wp] = fcn(p_d, dot_p_d, ddot_p_d, psi_d, p, dot_p, eta, Xip, hat_Wp)
m  = 1.82245;
g  = 9.81;
Ixx = 0.00749;
Ixy = -0.00051;
Ixz = -0.00003;
Iyy = 0.00978;
Iyz = -0.00098;
Izz = 0.05130;
gz      = [0; 0; g];
phi     = eta(1);
theta   = eta(2);
e_p     = p_d - p;
dot_e_p = dot_p_d - dot_p;
%% Position controller %%%
%%% Gains %%%
hat_m = 1*m; % mass uncertainty
KUp   = diag([4.5 4.5 9]);
Kip   = diag([0.5 0.5 0.8]);
Kp    = diag([1.8 1.8 1.8]);

Up       = dot_p_d + Kp*e_p;
dot_Up   = ddot_p_d + Kp*dot_e_p;
tilde_Up = Up - dot_p;
%%% Neural Network Structure %%%
gamma_p   = [1; dot_p; eta; dot_Up];
neurons_p = 10;
V_p = [0.6294   -0.0292    0.4863   -0.9311    0.3102    0.9186    0.2321   -0.8921   -0.6687    0.9923
    0.8116    0.6006   -0.2155   -0.1225   -0.6748    0.0944   -0.0534    0.0616    0.2040   -0.8436
   -0.7460   -0.7162    0.3110   -0.2369   -0.7620   -0.7228   -0.2967    0.5583   -0.4741   -0.1146
    0.8268   -0.1565   -0.6576    0.5310   -0.0033   -0.7014    0.6617    0.8680    0.3082   -0.7867
    0.2647    0.8315    0.4121    0.5904    0.9195   -0.4850    0.1705   -0.7402    0.3784    0.9238
   -0.8049    0.5844   -0.9363   -0.6263   -0.3192    0.6814    0.0994    0.1376    0.4963   -0.9907
   -0.4430    0.9190   -0.4462   -0.0205    0.1705   -0.4914    0.8344   -0.0612   -0.0989    0.5498
    0.0938    0.3115   -0.9077   -0.1088   -0.5524    0.6286   -0.4283   -0.9762   -0.8324    0.6346
    0.9150   -0.9286   -0.8057    0.2926    0.5025   -0.5130    0.5144   -0.3258   -0.5420    0.7374
    0.9298    0.6983    0.6469    0.4187   -0.4898    0.8585    0.5075   -0.6756    0.8267   -0.8311];
sigma_p = tanh(V_p'*gamma_p);
%%% Neural Network Gains %%%
flag_NN = 1; % <------------ On/Off NN
N_p     = 0.8*eye(neurons_p);   % 2   % 3.5 % 2.2  % 2.2 % 2.2  % 0.65
kp      = 0.4;                 % 0.1 % 0.4 % 1.25 % 1.2 % 1.15 % 0.001
a_p     = 0.001*diag([1 1 1]);
%%% Controller %%%
F_p        = KUp*tilde_Up + Kip*Xip + hat_m*(dot_Up + gz) + flag_NN*(hat_Wp'*sigma_p + a_p*sign(tilde_Up));
dot_hat_Wp = N_p*(sigma_p*tilde_Up' - kp*norm(tilde_Up)*hat_Wp);
theta_d    = atan((F_p(1)*cos(psi_d) + F_p(2)*sin(psi_d))/F_p(3));
phi_d      = atan(cos(theta_d)*(F_p(1)*sin(psi_d) - F_p(2)*cos(psi_d))/F_p(3));
F          = F_p(3)/(cos(phi)*cos(theta));
eta_d      = [phi_d; theta_d; psi_d];

== matlab function SURVEY_Simulations/Double two-loop (PID-Type + ANN)/NNC Orientation ==
  settings: updateMethod=DISCRETE
  data: eta_d input; tau output; tilde_Ueta output; dot_eta_d input; ddot_eta_d input; eta input; dot_eta input; Xieta input; hat_Weta input; dot_hat_Weta output; e_eta output
function [tau, tilde_Ueta, dot_hat_Weta, e_eta] = fcn(eta_d, dot_eta_d, ddot_eta_d, eta, dot_eta, Xieta, hat_Weta)

phi = eta(1) ; theta = eta(2);
%% Gains
K_Ueta = diag([0.5 0.5 1]);
K_ieta = diag([0.05 0.05 0.05]);
K_eta  = diag([4.8 4.8 8.5]);
%% Attitude Controller
e_eta     = eta_d - eta;
dot_e_eta = dot_eta_d - dot_eta;

Ueta       = dot_eta_d + K_eta*e_eta;
dot_Ueta   = ddot_eta_d + K_eta*dot_e_eta;
tilde_Ueta = Ueta - dot_eta;

gamma_eta = [1; eta; dot_eta; dot_Ueta; K_Ueta*tilde_Ueta];
neurons_eta = 10;
V_eta = [0.6294   -0.0292    0.4863   -0.9311    0.3102    0.9186    0.2321   -0.8921   -0.6687    0.9923
    0.8116    0.6006   -0.2155   -0.1225   -0.6748    0.0944   -0.0534    0.0616    0.2040   -0.8436
   -0.7460   -0.7162    0.3110   -0.2369   -0.7620   -0.7228   -0.2967    0.5583   -0.4741   -0.1146
    0.8268   -0.1565   -0.6576    0.5310   -0.0033   -0.7014    0.6617    0.8680    0.3082   -0.7867
    0.2647    0.8315    0.4121    0.5904    0.9195   -0.4850    0.1705   -0.7402    0.3784    0.9238
   -0.8049    0.5844   -0.9363   -0.6263   -0.3192    0.6814    0.0994    0.1376    0.4963   -0.9907
   -0.4430    0.9190   -0.4462   -0.0205    0.1705   -0.4914    0.8344   -0.0612   -0.0989    0.5498
    0.0938    0.3115   -0.9077   -0.1088   -0.5524    0.6286   -0.4283   -0.9762   -0.8324    0.6346
    0.9150   -0.9286   -0.8057    0.2926    0.5025   -0.5130    0.5144   -0.3258   -0.5420    0.7374
    0.9298    0.6983    0.6469    0.4187   -0.4898    0.8585    0.5075   -0.6756    0.8267   -0.8311
   -0.6848    0.8680    0.3897    0.5094    0.0119   -0.3000   -0.2391    0.5886   -0.6952   -0.2004
    0.9412    0.3575   -0.3658   -0.4479    0.3982   -0.6068    0.1356   -0.3776    0.6516   -0.4803
    0.9143    0.5155    0.9004    0.3594    0.7818   -0.4978   -0.8483    0.0571    0.0767    0.6001];

sigma_eta = tanh(V_eta'*gamma_eta);
N_eta = 1.15*eye(neurons_eta);% 22  % 22   % 12   % 30
keta  = 0.15;                % 3.9 % 3.95 % 3.95 % 3.95
a_eta = 0.001*diag([1 1 1]);

W = [1  sin(phi)*tan(theta)  cos(phi)*tan(theta)
     0  cos(phi)             -sin(phi)
     0  sin(phi)/cos(theta)  cos(phi)/cos(theta)];

tau_eta = K_Ueta*tilde_Ueta + K_ieta*Xieta + hat_Weta'*sigma_eta + a_eta*sign(tilde_Ueta);
tau     = W'*tau_eta;
dot_hat_Weta = N_eta*(sigma_eta*tilde_Ueta' - keta*norm(tilde_Ueta)*hat_Weta);

== matlab function SURVEY_Simulations/Subsystem2/MATLAB Function ==
  data: F input; ddot_p output; ddot_eta output; tau input; delta_p input; delta_eta input; dot_p input; eta input; dot_eta input
function [ddot_p, ddot_eta] = fcn(F, tau, delta_p, delta_eta, dot_p, eta, dot_eta)

m  = 1.82245;
g  = 9.81;
Ixx = 0.00749;
Ixy = -0.00051;
Ixz = -0.00003;
Iyy = 0.00978;
Iyz = -0.00098;
Izz = 0.05130;
dx = 0.002; dy = 0.002; dz = 0.004;
d_phi = 0.002; d_theta = 0.002; d_psi = 0.004;

I  = [Ixx Ixy Ixz
      Ixy Iyy Iyz
      Ixz Iyz Izz];
Dp = diag([dx dy dz]);
Dn = diag([d_phi d_theta d_psi]);
Vz = [0; 0; 1];

phi     = eta(1);     theta     = eta(2);     psi = eta(3);
dot_phi = dot_eta(1); dot_theta = dot_eta(2);

R = [cos(theta)*cos(psi)  sin(phi)*sin(theta)*cos(psi)-cos(phi)*sin(psi)  cos(phi)*sin(theta)*cos(psi)+sin(phi)*sin(psi)
     cos(theta)*sin(psi)  sin(phi)*sin(theta)*sin(psi)+cos(phi)*cos(psi)  cos(phi)*sin(theta)*sin(psi)-sin(phi)*cos(psi)
     -sin(theta)          sin(phi)*cos(theta)                             cos(phi)*cos(theta)];
 
% W = [1  sin(phi)*tan(theta)  cos(phi)*tan(theta)
%      0  cos(phi)             -sin(phi)
%      0  sin(phi)/cos(theta)  cos(phi)/cos(theta)];

iW = [1 0         -sin(theta)
      0 cos(phi)  cos(theta)*sin(phi)
      0 -sin(phi) cos(theta)*cos(phi)];
 
dot_W = [0  (cos(phi)*tan(theta))+((sin(phi)*dot_theta)/(cos(theta)^2))                     ((cos(phi)*dot_theta)/(cos(theta)^2))-(sin(phi)*tan(theta)*dot_phi)
         0  -sin(phi)*dot_phi                                                               -cos(phi)*dot_phi
         0  ((cos(phi)*cos(theta)*dot_phi)+(sin(phi)*sin(theta)*dot_theta))/(cos(theta)^2)  ((cos(phi)*sin(theta)*dot_theta)-(sin(phi)*cos(theta)*dot_phi))/(cos(theta)^2)];
  
iWdot_eta = iW*dot_eta;

SiWdot_eta = [0              -iWdot_eta(3)  iWdot_eta(2)
              iWdot_eta(3)   0              -iWdot_eta(1)
              -iWdot_eta(2)  iWdot_eta(1)   0];

M = iW'*I*iW;
C = iW'*(SiWdot_eta*I - I*iW*dot_W)*iW;

ddot_p   = (R*Vz*F + delta_p - m*g*Vz - Dp*dot_p)/m;
ddot_eta = M\(iW'*tau + delta_eta - C*dot_eta - Dn*dot_eta);

== matlab function SURVEY_Simulations/Model-free linear PID/MATLAB Function1 ==
  data: eeta input; tau output; dot_eeta input; int_eeta input
function tau = fcn(eeta, dot_eeta, int_eeta)
Kpeta = diag([4.5 4.5 6.5]);
Kdeta = diag([1.75 1.75 3.75]);
Kieta = diag([0.5 0.5 0.5]);

tau = Kpeta*eeta + Kdeta*dot_eeta + Kieta*int_eeta;

== matlab function SURVEY_Simulations/QBall 2 Quadrotor 4/MATLAB Function ==
  data: F input; ddot_p output; ddot_eta output; tau input; delta_p input; delta_eta input; dot_p input; eta input; dot_eta input
function [ddot_p, ddot_eta] = fcn(F, tau, delta_p, delta_eta, dot_p, eta, dot_eta)

m  = 1.82245;
g  = 9.81;
Ixx = 0.00749;
Ixy = -0.00051;
Ixz = -0.00003;
Iyy = 0.00978;
Iyz = -0.00098;
Izz = 0.05130;
dx = 0.002; dy = 0.002; dz = 0.004;
d_phi = 0.002; d_theta = 0.002; d_psi = 0.004;
I  = [Ixx Ixy Ixz
      Ixy Iyy Iyz
      Ixz Iyz Izz];
Dp = diag([dx dy dz]);
Dn = diag([d_phi d_theta d_psi]);
Vz = [0; 0; 1];

phi     = eta(1);     theta     = eta(2);     psi = eta(3);
dot_phi = dot_eta(1); dot_theta = dot_eta(2);

R = [cos(theta)*cos(psi)  sin(phi)*sin(theta)*cos(psi)-cos(phi)*sin(psi)  cos(phi)*sin(theta)*cos(psi)+sin(phi)*sin(psi)
     cos(theta)*sin(psi)  sin(phi)*sin(theta)*sin(psi)+cos(phi)*cos(psi)  cos(phi)*sin(theta)*sin(psi)-sin(phi)*cos(psi)
     -sin(theta)          sin(phi)*cos(theta)                             cos(phi)*cos(theta)];
 
% W = [1  sin(phi)*tan(theta)  cos(phi)*tan(theta)
%      0  cos(phi)             -sin(phi)
%      0  sin(phi)/cos(theta)  cos(phi)/cos(theta)];

iW = [1 0         -sin(theta)
      0 cos(phi)  cos(theta)*sin(phi)
      0 -sin(phi) cos(theta)*cos(phi)];
 
dot_W = [0  (cos(phi)*tan(theta))+((sin(phi)*dot_theta)/(cos(theta)^2))                     ((cos(phi)*dot_theta)/(cos(theta)^2))-(sin(phi)*tan(theta)*dot_phi)
         0  -sin(phi)*dot_phi                                                               -cos(phi)*dot_phi
         0  ((cos(phi)*cos(theta)*dot_phi)+(sin(phi)*sin(theta)*dot_theta))/(cos(theta)^2)  ((cos(phi)*sin(theta)*dot_theta)-(sin(phi)*cos(theta)*dot_phi))/(cos(theta)^2)];
  
iWdot_eta = iW*dot_eta;

SiWdot_eta = [0              -iWdot_eta(3)  iWdot_eta(2)
              iWdot_eta(3)   0              -iWdot_eta(1)
              -iWdot_eta(2)  iWdot_eta(1)   0];

M = iW'*I*iW;
C = iW'*(SiWdot_eta*I - I*iW*dot_W)*iW;

ddot_p   = (R*Vz*F + delta_p - m*g*Vz - Dp*dot_p)/m;
ddot_eta = M\(iW'*tau + delta_eta - C*dot_eta - Dn*dot_eta);

== matlab function SURVEY_Simulations/QBall 2 Quadrotor 1/MATLAB Function ==
  data: F input; ddot_p output; ddot_eta output; tau input; delta_p input; delta_eta input; dot_p input; eta input; dot_eta input
function [ddot_p, ddot_eta] = fcn(F, tau, delta_p, delta_eta, dot_p, eta, dot_eta)

m  = 1.82245;
g  = 9.81;
Ixx = 0.00749;
Ixy = -0.00051;
Ixz = -0.00003;
Iyy = 0.00978;
Iyz = -0.00098;
Izz = 0.05130;
dx = 0.002; dy = 0.002; dz = 0.004;
d_phi = 0.002; d_theta = 0.002; d_psi = 0.004;
I  = [Ixx Ixy Ixz
      Ixy Iyy Iyz
      Ixz Iyz Izz];
Dp = diag([dx dy dz]);
Dn = diag([d_phi d_theta d_psi]);
Vz = [0; 0; 1];

phi     = eta(1);     theta     = eta(2);     psi = eta(3);
dot_phi = dot_eta(1); dot_theta = dot_eta(2);

R = [cos(theta)*cos(psi)  sin(phi)*sin(theta)*cos(psi)-cos(phi)*sin(psi)  cos(phi)*sin(theta)*cos(psi)+sin(phi)*sin(psi)
     cos(theta)*sin(psi)  sin(phi)*sin(theta)*sin(psi)+cos(phi)*cos(psi)  cos(phi)*sin(theta)*sin(psi)-sin(phi)*cos(psi)
     -sin(theta)          sin(phi)*cos(theta)                             cos(phi)*cos(theta)];
 
% W = [1  sin(phi)*tan(theta)  cos(phi)*tan(theta)
%      0  cos(phi)             -sin(phi)
%      0  sin(phi)/cos(theta)  cos(phi)/cos(theta)];

iW = [1 0         -sin(theta)
      0 cos(phi)  cos(theta)*sin(phi)
      0 -sin(phi) cos(theta)*cos(phi)];
 
dot_W = [0  (cos(phi)*tan(theta))+((sin(phi)*dot_theta)/(cos(theta)^2))                     ((cos(phi)*dot_theta)/(cos(theta)^2))-(sin(phi)*tan(theta)*dot_phi)
         0  -sin(phi)*dot_phi                                                               -cos(phi)*dot_phi
         0  ((cos(phi)*cos(theta)*dot_phi)+(sin(phi)*sin(theta)*dot_theta))/(cos(theta)^2)  ((cos(phi)*sin(theta)*dot_theta)-(sin(phi)*cos(theta)*dot_phi))/(cos(theta)^2)];
  
iWdot_eta = iW*dot_eta;

SiWdot_eta = [0              -iWdot_eta(3)  iWdot_eta(2)
              iWdot_eta(3)   0              -iWdot_eta(1)
              -iWdot_eta(2)  iWdot_eta(1)   0];

M = iW'*I*iW;
C = iW'*(SiWdot_eta*I - I*iW*dot_W)*iW;

ddot_p   = (R*Vz*F + delta_p - m*g*Vz - Dp*dot_p)/m;
ddot_eta = M\(iW'*tau + delta_eta - C*dot_eta - Dn*dot_eta);

== matlab function SURVEY_Simulations/Nonlinear PI//PID regulation/MATLAB Function ==
  data: tilde_qu input; tilde_qa input; F output; dot_tilde_qa input; dot_tilde_qu input; int_tilde_qu input; int_tilde_qa input; eta input; tau output; phi_d output; theta_d output
function [F, tau, phi_d, theta_d] = fcn(tilde_qu, tilde_qa, dot_tilde_qa, dot_tilde_qu, int_tilde_qu, int_tilde_qa, eta)

m = 1.82245;
g = 9.81;

Kpa = diag([15 5 5 5]);
Kda = diag([9 3.5 3.5 3.5]);
Kia = diag([0.2 0.5 0.5 0.5]);

beta = 1;
Kpu = diag([0.85 0.85]);
Kdu = diag([0.5 0.5]);
Kiu = diag([0.05 0.05]);

phi   = eta(1);
theta = eta(2);
psi   = eta(3);

%------------- Actuated part
R = [cos(theta)*cos(psi)  sin(phi)*sin(theta)*cos(psi)-cos(phi)*sin(psi)  cos(phi)*sin(theta)*cos(psi)+sin(phi)*sin(psi)
     cos(theta)*sin(psi)  sin(phi)*sin(theta)*sin(psi)+cos(phi)*cos(psi)  cos(phi)*sin(theta)*sin(psi)-sin(phi)*cos(psi)
     -sin(theta)          sin(phi)*cos(theta)                             cos(phi)*cos(theta)];

% W = [1  sin(phi)*tan(theta)  cos(phi)*tan(theta)
%      0  cos(phi)             -sin(phi)
%      0  sin(phi)/cos(theta)  cos(phi)/cos(theta)];

iW = [1 0         -sin(theta)
      0 cos(phi)  cos(theta)*sin(phi)
      0 -sin(phi) cos(theta)*cos(phi)];

iWT = iW';

ga = [m*g; 0; 0; 0];

Ba = [R(3,3) 0        0        0
      0      iWT(1,1) iWT(1,2) iWT(1,3)
      0      iWT(2,1) iWT(2,2) iWT(2,3)
      0      iWT(3,1) iWT(3,2) iWT(3,3)];

U_a = Ba\(Kpa*tilde_qa + Kda*dot_tilde_qa + Kia*int_tilde_qa + ga);

%------------ Underactuated part
A_qa = [sin(psi)              -cos(psi)
        1/(cos(phi)*cos(psi)) 0];

a_qa = [0; -tan(phi)*tan(psi)];

Xi = beta*A_qa*(Kpu*tilde_qu + Kiu*int_tilde_qu + Kdu*dot_tilde_qu) + a_qa;

phi_d   = asin(Xi(1));
theta_d = asin(Xi(2));

Bu = [R(1,3) 0
      0      R(2,3)];

F = U_a(1);
tau = [U_a(2); U_a(3); U_a(4)];

== matlab function SURVEY_Simulations/QBall 2 Quadrotor 2/MATLAB Function ==
  data: F input; ddot_p output; ddot_eta output; tau input; delta_p input; delta_eta input; dot_p input; eta input; dot_eta input
function [ddot_p, ddot_eta] = fcn(F, tau, delta_p, delta_eta, dot_p, eta, dot_eta)

m  = 1.82245;
g  = 9.81;
Ixx = 0.00749;
Ixy = -0.00051;
Ixz = -0.00003;
Iyy = 0.00978;
Iyz = -0.00098;
Izz = 0.05130;
dx = 0.002; dy = 0.002; dz = 0.004;
d_phi = 0.002; d_theta = 0.002; d_psi = 0.004;
I  = [Ixx Ixy Ixz
      Ixy Iyy Iyz
      Ixz Iyz Izz];
Dp = diag([dx dy dz]);
Dn = diag([d_phi d_theta d_psi]);
Vz = [0; 0; 1];

phi     = eta(1);     theta     = eta(2);     psi = eta(3);
dot_phi = dot_eta(1); dot_theta = dot_eta(2);

R = [cos(theta)*cos(psi)  sin(phi)*sin(theta)*cos(psi)-cos(phi)*sin(psi)  cos(phi)*sin(theta)*cos(psi)+sin(phi)*sin(psi)
     cos(theta)*sin(psi)  sin(phi)*sin(theta)*sin(psi)+cos(phi)*cos(psi)  cos(phi)*sin(theta)*sin(psi)-sin(phi)*cos(psi)
     -sin(theta)          sin(phi)*cos(theta)                             cos(phi)*cos(theta)];
 
% W = [1  sin(phi)*tan(theta)  cos(phi)*tan(theta)
%      0  cos(phi)             -sin(phi)
%      0  sin(phi)/cos(theta)  cos(phi)/cos(theta)];

iW = [1 0         -sin(theta)
      0 cos(phi)  cos(theta)*sin(phi)
      0 -sin(phi) cos(theta)*cos(phi)];
 
dot_W = [0  (cos(phi)*tan(theta))+((sin(phi)*dot_theta)/(cos(theta)^2))                     ((cos(phi)*dot_theta)/(cos(theta)^2))-(sin(phi)*tan(theta)*dot_phi)
         0  -sin(phi)*dot_phi                                                               -cos(phi)*dot_phi
         0  ((cos(phi)*cos(theta)*dot_phi)+(sin(phi)*sin(theta)*dot_theta))/(cos(theta)^2)  ((cos(phi)*sin(theta)*dot_theta)-(sin(phi)*cos(theta)*dot_phi))/(cos(theta)^2)];
  
iWdot_eta = iW*dot_eta;

SiWdot_eta = [0              -iWdot_eta(3)  iWdot_eta(2)
              iWdot_eta(3)   0              -iWdot_eta(1)
              -iWdot_eta(2)  iWdot_eta(1)   0];

M = iW'*I*iW;
C = iW'*(SiWdot_eta*I - I*iW*dot_W)*iW;

ddot_p   = (R*Vz*F + delta_p - m*g*Vz - Dp*dot_p)/m;
ddot_eta = M\(iW'*tau + delta_eta - C*dot_eta - Dn*dot_eta);

== matlab function SURVEY_Simulations/Model Based Controller/MBC Orientation ==
  data: eta_d input; tau output; tilde_Ueta output; dot_eta_d input; ddot_eta_d input; eta input; dot_eta input; e_eta output; Xieta input
function [tau,tilde_Ueta, e_eta] = fcn(eta_d, dot_eta_d, ddot_eta_d, eta, dot_eta,  Xieta)

phi     = eta(1);     theta = eta(2);
dot_phi = dot_eta(1); dot_theta = dot_eta(2);
Ixx = 0.00749;
Iyy = 0.00978;
Izz = 0.05130;
d_phi = 0.002; d_theta = 0.002; d_psi = 0.004;
I  = diag([Ixx Iyy Izz]);
Dn = diag([d_phi d_theta d_psi]);
%% Gains
K1eta = diag([0.5 0.5 1]);
K2eta = diag([0.05 0.05 0.05]);
K3eta = diag([4.8 4.8 8.5]);

e_eta     = eta_d - eta;
dot_e_eta = dot_eta_d - dot_eta;

Ueta     = dot_eta_d + K3eta*e_eta;
dot_Ueta = ddot_eta_d + K3eta*dot_e_eta;

tilde_Ueta = Ueta - dot_eta;

W = [1  sin(phi)*tan(theta)  cos(phi)*tan(theta)
     0  cos(phi)             -sin(phi)
     0  sin(phi)/cos(theta)  cos(phi)/cos(theta)];

iW = [1 0         -sin(theta)
      0 cos(phi)  cos(theta)*sin(phi)
      0 -sin(phi) cos(theta)*cos(phi)];
 
dot_W = [0  (cos(phi)*tan(theta))+((sin(phi)*dot_theta)/(cos(theta)^2))                     ((cos(phi)*dot_theta)/(cos(theta)^2))-(sin(phi)*tan(theta)*dot_phi)
         0  -sin(phi)*dot_phi                                                               -cos(phi)*dot_phi
         0  ((cos(phi)*cos(theta)*dot_phi)+(sin(phi)*sin(theta)*dot_theta))/(cos(theta)^2)  ((cos(phi)*sin(theta)*dot_theta)-(sin(phi)*cos(theta)*dot_phi))/(cos(theta)^2)];
  
iWdot_eta = iW*dot_eta;

SiWdot_eta = [0              -iWdot_eta(3)  iWdot_eta(2)
              iWdot_eta(3)   0              -iWdot_eta(1)
              -iWdot_eta(2)  iWdot_eta(1)   0];

M = iW'*I*iW;
C = iW'*(SiWdot_eta*I - I*iW*dot_W)*iW;
tau = W'*(K1eta*tilde_Ueta + K2eta*Xieta + M*dot_Ueta + (C + Dn)*dot_eta);

== matlab function SURVEY_Simulations/Subsystem1/MATLAB Function ==
  data: F input; ddot_p output; ddot_eta output; tau input; delta_p input; delta_eta input; dot_p input; eta input; dot_eta input
function [ddot_p, ddot_eta] = fcn(F, tau, delta_p, delta_eta, dot_p, eta, dot_eta)

m  = 1.82245;
g  = 9.81;
Ixx = 0.00749;
Ixy = -0.00051;
Ixz = -0.00003;
Iyy = 0.00978;
Iyz = -0.00098;
Izz = 0.05130;
dx = 0.002; dy = 0.002; dz = 0.004;
d_phi = 0.002; d_theta = 0.002; d_psi = 0.004;

I  = [Ixx Ixy Ixz
      Ixy Iyy Iyz
      Ixz Iyz Izz];
Dp = diag([dx dy dz]);
Dn = diag([d_phi d_theta d_psi]);
Vz = [0; 0; 1];

phi     = eta(1);     theta     = eta(2);     psi = eta(3);
dot_phi = dot_eta(1); dot_theta = dot_eta(2);

R = [cos(theta)*cos(psi)  sin(phi)*sin(theta)*cos(psi)-cos(phi)*sin(psi)  cos(phi)*sin(theta)*cos(psi)+sin(phi)*sin(psi)
     cos(theta)*sin(psi)  sin(phi)*sin(theta)*sin(psi)+cos(phi)*cos(psi)  cos(phi)*sin(theta)*sin(psi)-sin(phi)*cos(psi)
     -sin(theta)          sin(phi)*cos(theta)                             cos(phi)*cos(theta)];
 
% W = [1  sin(phi)*tan(theta)  cos(phi)*tan(theta)
%      0  cos(phi)             -sin(phi)
%      0  sin(phi)/cos(theta)  cos(phi)/cos(theta)];

iW = [1 0         -sin(theta)
      0 cos(phi)  cos(theta)*sin(phi)
      0 -sin(phi) cos(theta)*cos(phi)];
 
dot_W = [0  (cos(phi)*tan(theta))+((sin(phi)*dot_theta)/(cos(theta)^2))                     ((cos(phi)*dot_theta)/(cos(theta)^2))-(sin(phi)*tan(theta)*dot_phi)
         0  -sin(phi)*dot_phi                                                               -cos(phi)*dot_phi
         0  ((cos(phi)*cos(theta)*dot_phi)+(sin(phi)*sin(theta)*dot_theta))/(cos(theta)^2)  ((cos(phi)*sin(theta)*dot_theta)-(sin(phi)*cos(theta)*dot_phi))/(cos(theta)^2)];
  
iWdot_eta = iW*dot_eta;

SiWdot_eta = [0              -iWdot_eta(3)  iWdot_eta(2)
              iWdot_eta(3)   0              -iWdot_eta(1)
              -iWdot_eta(2)  iWdot_eta(1)   0];

M = iW'*I*iW;
C = iW'*(SiWdot_eta*I - I*iW*dot_W)*iW;

ddot_p   = (R*Vz*F + delta_p - m*g*Vz - Dp*dot_p)/m;
ddot_eta = M\(iW'*tau + delta_eta - C*dot_eta - Dn*dot_eta);

== matlab function SURVEY_Simulations/Model Based Controller/MBC Position ==
  data: p_d input; F output; tilde_Up output; dot_p_d input; ddot_p_d input; p input; dot_p input; eta input; psi_d input; eta_d output; Xip input
function [F, tilde_Up, eta_d] = fcn(p_d, dot_p_d, ddot_p_d, p, dot_p, eta, psi_d, Xip)
m  = 1.82245;
g  = 9.81;
gz = [0; 0; g];
dx = 0.002; dy = 0.002; dz = 0.004;
Dp = diag([dx dy dz]);
phi = eta(1) ; theta = eta(2);

e_p     = p_d - p;
dot_e_p = dot_p_d - dot_p;
%% Position Controller
%Gains
K1p = diag([4.5 4.5 9]);
K2p = diag([0.5 0.5 0.8]);
K3p = diag([1.8 1.8 1.8]);

Up       = dot_p_d + K3p*e_p;
dot_Up   = ddot_p_d + K3p*dot_e_p;
tilde_Up = Up - dot_p;

F_p     = K1p*tilde_Up + K2p*Xip + m*(dot_Up + gz) + Dp*dot_p;
theta_d = atan((F_p(1)*cos(psi_d) + F_p(2)*sin(psi_d))/F_p(3));
phi_d   = atan(cos(theta_d)*(F_p(1)*sin(psi_d) - F_p(2)*cos(psi_d))/F_p(3));
F       = F_p(3)/(cos(phi)*cos(theta));

eta_d = [phi_d; theta_d; psi_d];
